simulink model "test11"  (R2021a)
settings: Solver=VariableStepAuto  StartTime=0.0  StopTime=8  RelTol=1e-3
model workspace (MAT data in the model file):
  SDO_OutputTimes = [0 0.00347222222222 0.00694444444444 0.0104166666667 0.0138888888889 0.0173611111111 0.0208333333333 0.0243055555556 0.0277777777778 0.03125 0.0347222222222 0.0381944444444 ... (4607 elements, 4607x1)]
  params : climate_p (value not decoded)
libraries: HORTISIM x3
(part 2 of 2)

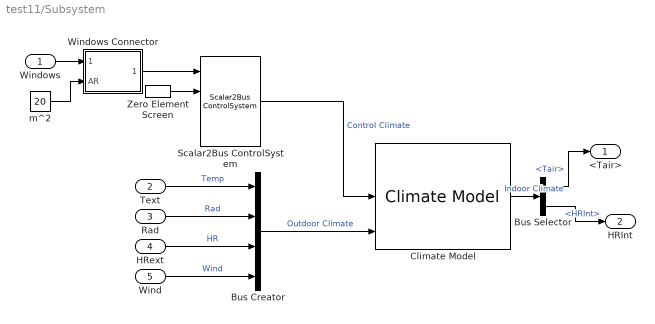
== system test11/Subsystem ==
  Windows : Inport
  Text : Inport  Port=2
  Rad : Inport  Port=3
  HRext : Inport  Port=4
  Wind : Inport  Port=5
  Bus Creator : BusCreator  Inputs=4
  Bus Selector : BusSelector  OutputSignals=Temp.Tair,Gas.HRInt
  Climate Model : HORTISIM/Climate/Models/Climate Model  params=params  x0=cic
      settings: SourceProductName=Horti Simulator
  Scalar2Bus ControlSystem : HORTISIM/Other  Functions/Scalar2Bus  ControlSystem  SystemSampleTime=-1  VariantActivationTime=update diagram  Latency=0  AutoFrameSizeCalculation=off
      settings: SourceProductName=Horti Simulator
  Windows Connector : Subsystem
  Zero Element Screen : HORTISIM/Other  Functions/Zero Element Screen  SystemSampleTime=-1  VariantActivationTime=update diagram  Latency=0  AutoFrameSizeCalculation=off
      settings: SourceProductName=Horti Simulator
  m^2 : Constant  Value=20
  <Tair> : Outport
  HRInt : Outport  Port=2
  wires:
  Scalar2Bus ControlSystem/1 -> Climate Model/2  "Control Climate"
  Climate Model/1 -> Bus Selector/1  "Indoor Climate"
  Bus Creator/1 -> Climate Model/3  "Outdoor Climate"
  Bus Selector/1 -> <Tair>/1  "<Tair>"
  Rad/1 -> Bus Creator/2  "Rad"
  HRext/1 -> Bus Creator/3  "HR"
  Wind/1 -> Bus Creator/4  "Wind"
  Text/1 -> Bus Creator/1  "Temp"
  Bus Selector/2 -> HRInt/1  "<HRInt>"
  Zero Element Screen/1 -> Scalar2Bus ControlSystem/2
  Windows/1 -> Windows Connector/1(value)
  m^2/1 -> Windows Connector/2(AR)
  Windows Connector/1(Windows) -> Scalar2Bus ControlSystem/1

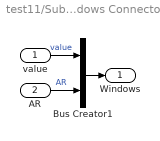
== system test11/Subsystem/Windows Connector ==
  value : Inport
  AR : Inport  Port=2
  Bus Creator1 : BusCreator  Inputs=2
  Windows : Outport
  wires:
  Bus Creator1/1 -> Windows/1
  value/1 -> Bus Creator1/1  "value"
  AR/1 -> Bus Creator1/2  "AR"
